simulink model "ComputedTorqueControl"  (R2020a)
settings: Solver=VariableStepAuto  StartTime=0.0  StopTime=1.5  RelTol=1e-3
values from neighbouring files (symbols this model uses):
  ADAMS_communication_interval = 0.005    [ControlsPlantTorqueControl.m]
  ADAMS_communications_per_output_step = 1    [ControlsPlantTorqueControl.m]
  ADAMS_cwd = 'C:\Users\Gowri Umesh\OneDrive\Desktop\RAJEEV_UMESH_AMORO_Report\ComputedTorqueControl'    [ControlsPlantTorqueControl.m]
  ADAMS_exec = ''    [ControlsPlantTorqueControl.m]
  ADAMS_host = 'DESKTOP-1FI5JCT'    [ControlsPlantTorqueControl.m]
  ADAMS_init = ''    [ControlsPlantTorqueControl.m]
  ADAMS_inputs = 'f1!f2'    [ControlsPlantTorqueControl.m]
  ADAMS_outputs = 'q1!q2'    [ControlsPlantTorqueControl.m]
  ADAMS_prefix = 'ControlsPlantTorqueControl'    [ControlsPlantTorqueControl.m]
  ADAMS_static = 'no'    [ControlsPlantTorqueControl.m]
  ADAMS_sysdir = 'C:\PROGRA~1\MSC~1.SOF\ADAMSS~1\2020_1\'    [ControlsPlantTorqueControl.m]
  ADAMS_time_offset = 0.0    (= 0)    [ControlsPlantTorqueControl.m]
settings Model: Creator=Gowri Umesh  LastModifiedBy=Gowri Umesh
settings DebuggingCC: AlgebraicLoopMsg=none

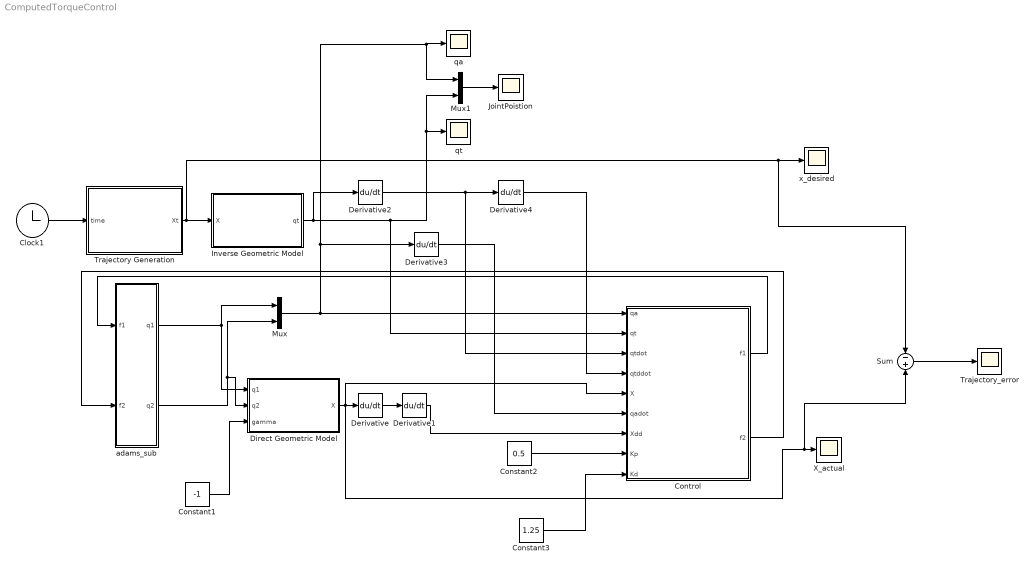
== system ComputedTorqueControl ==
  Clock1 : Clock
  Constant1 : Constant  Value=-1
  Constant2 : Constant  Value=0.5
  Constant3 : Constant  Value=1.25
  Control : MATLAB Function  TreatAsAtomicUnit=on
  Derivative{,1..4} (5 alike) : Derivative
  Direct Geometric Model : MATLAB Function  TreatAsAtomicUnit=on
  Inverse Geometric Model : MATLAB Function  TreatAsAtomicUnit=on
  JointPoistion : Scope
  Mux : Mux  Inputs=2
  Mux1 : Mux  Inputs=2
  Sum : Sum  Inputs=-+
  Trajectory Generation : MATLAB Function  TreatAsAtomicUnit=on
  Trajectory_error : Scope
  X_actual : Scope
  adams_sub : Subsystem
  qa : Scope
  qt : Scope
  x_desired : Scope
  wires:
  Sum/1 -> Trajectory_error/1
  Control/1(f1) -> adams_sub/1(f1)
  Control/2(f2) -> adams_sub/2(f2)
  Constant1/1 -> Direct Geometric Model/3(gamma)
  adams_sub/1(q1) -> Direct Geometric Model/1(q1), Mux/1
  adams_sub/2(q2) -> Mux/2, Direct Geometric Model/2(q2)
  Clock1/1 -> Trajectory Generation/1(time)
  Derivative/1 -> Derivative1/1
  Trajectory Generation/1(Xt) -> Sum/1, x_desired/1, Inverse Geometric Model/1(X)
  Mux/1 -> Mux1/1, qa/1, Derivative3/1, Control/1(qa)
  Inverse Geometric Model/1(qt) -> Derivative2/1, Mux1/2, qt/1, Control/2(qt)
  Derivative2/1 -> Control/3(qtdot), Derivative4/1
  Derivative3/1 -> Control/6(qadot)
  Direct Geometric Model/1(X) -> Control/5(X), Derivative/1, Sum/2, X_actual/1
  Derivative1/1 -> Control/7(Xdd)
  Derivative4/1 -> Control/4(qtddot)
  Constant2/1 -> Control/8(Kp)
  Constant3/1 -> Control/9(Kd)
  Mux1/1 -> JointPoistion/1

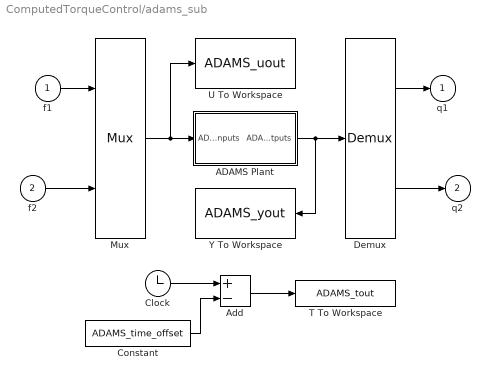
== system ComputedTorqueControl/adams_sub ==
  f1 : Inport
  f2 : Inport  Port=2
  ADAMS Plant : Subsystem  LoadFcn=|  InitFcn=clear mex  mask(Adams Plant){exevie=ADAMS_sysdir, nam_in=ADAMS_inputs, namout=ADAMS_outputs, nampre=ADAMS_prefix, outfil=ADAMS_prefix, exesol=ADAMS_exec, stat=ADAMS_static, inicmd=[ADAMS_init], exetyp=C++, comtyp=PIPE(DDE), workdir=ADAMS_cwd, ada_host=ADAMS_host, modani=batch, modsim=discrete, dft=no, simulink_lead_cosim=yes, pin_interp_order=0, pout_extrap_order=0, pin_extrap_order=0, pout_interp_order=0, dt_out=ADAMS_communication_interval, o_rate=ADAMS_communications_per_output_step, time_offset=ADAMS_time_offset, more=off}
      | %check based on dialog box setting for when setting by popup menu                                             
      | if exist('ADAMS_solver_type')                                                                                 
      |   if strcmp(ADAMS_solver_type,'C++')                                                                          
      |     set_param(gcb,'exetyp','C++');                                                                            
      |   else                                                                                                        
      |     set_param(gcb,'exetyp','Fortran');                                                                        
      |   end                                                                                                         
      | else                                                                                                          
      |   set_param(gcb,'exetyp','C++');                                                                              
      | end                                                                                                           
      | %set the mode if using acar_solver                                                                            
      | %REQUIRED HERE BECAUSE BELOW CAUSES MDLTERMINATE TO BE CALLED 2 TIMES IN MIDDLE OF SIMULATION WHEN SET IN MASK
      |                                                                                                               
      | %enable the direct feedthrough, sim mode, anim mode parameters by default                                     
      |                                                                                                               
      | if exist('set_some_params_states')                                                                            
      |                                                                                                               
      |   set_some_params_states({'dft','modsim','modani'},{'on','on','on'},'MaskEnables',gcb)                        
      |   %turn on direct feedthrough option                                                                          
      |   set_some_params_states({'dft'},{'on'},'MaskVisibilities',gcb)                                               
      |                                                                                                               
      |  end                                                                                                          
      |                                                                                                               
      |                                                                                                               
      | if exist('ADAMS_exec')                                                                                        
      |   if and(strcmp(get_param(gcb,'exesol'),'ADAMS_exec'),strcmp(ADAMS_exec,'acar_solver'))                       
      |     %set the sim mode to discrete -- only supported mode                                                      
      |     set_param(gcb,'modsim','discrete')                                                                        
      |      %turn off direct feedthrough option                                                                      
      |      set_some_params_states({'dft'},{'off'},'MaskVisibilities',gcb)                                           
      |     %set the animation mode to batch -- only supported mode                                                   
      |     set_param(gcb,'modani','batch')                                                                           
      |     %disable the direct feedthrough, sim mode, anim mode parameters                                           
      |     set_some_params_states({'modsim','modani'},{'off','off'},'MaskEnables',gcb)                               
      |   end
      |   if and(strcmp(get_param(gcb,'exesol'),'ADAMS_exec'),strcmp(ADAMS_exec,'apre_solver'))                       
      |     %set the sim mode to discrete -- only supported mode                                                      
      |     set_param(gcb,'modsim','discrete')                                                                        
      |      %turn off direct feedthrough option                                                                      
      |      set_some_params_states({'dft'},{'off'},'MaskVisibilities',gcb)                                           
      |     %set the animation mode to batch -- only supported mode                                                   
      |     set_param(gcb,'modani','batch')                                                                           
      |     %disable the direct feedthrough, sim mode, anim mode parameters                                           
      |     set_some_params_states({'modsim','modani'},{'off','off'},'MaskEnables',gcb)                               
      |   end                                                                                                  
      | end
      mask prompts: exevie "Adams install directory"; nam_in "Adams View input names"; namout "Adams View output names"; nampre "Adams model file prefix"; outfil "Output files prefix (opt.: if blank - no output)"; exesol "User executable (opt.: if blank - use standard)"; stat "Initial static simulation flag"; inicmd "Initialization commands"; exetyp "Adams Solver type"; comtyp "Interprocess option"; workdir "Adams working directory"; ada_host "Adams host"; modani "Animation mode"; modsim "Simulation mode"; dft "Direct feedthrough"; simulink_lead_cosim "Discrete Computational Order - Simulink Leads Adams"; pin_interp_order "Plant input interpolation order"; pout_extrap_order "Plant output extrapolation order"; pin_extrap_order "Plant input extrapolation order"; pout_interp_order "Plant output interpolation order"; dt_out "Communication interval"; o_rate "Number of communications per output step"; time_offset "Offset between Simulink and Adams simulation time"; more "More parameters"
      mask help: Simulate any Adams plant model either in Adams Solver form (.adm file) or in Adams View form (.cmd file)
      settings: OpenFcn=|
      | open_system(gcb,'mask')
      | if not(exist('set_some_params_states'))
      | 
      | warning('The script "set_some_params_states.m" cannot be found in the MATLAB PATH.  Cannot update the ADAMS Plant S-Function parameters.')
      | 
      | warning('Recommended action(optional):  run the Adams Controls .m file first to help choose the correct settings in the Adams S-Function block.')
      | 
      | end
      mask Help:
      | <html>
      | This S-Function represents the non-linear Adams Plant with the inputs sent to the Adams model as input #1 and Time as input #2<br>
      |  and the outputs generated by the Adams model.  See the Adams Controls documentation for more <br>
      | information.  This plant uses the following variables:<br>
      | <br>
      | <b>ADAMS_sysdir:</b> Adams installation directory<br>
      | <b>ADAMS_inputs:</b> Input variables View names vector<br>
      | <b>ADAMS_outputs :</b> Outputs variables View names vector<br>
      | <b>ADAMS_prefix:</b> ADAMS model files prefix (.adm, .cmd); also doubles as output files prefix<br>
      | <b>ADAMS_exec:</b>  Adams Solver user library or keyword (e.g., acar_solver)<br>
      | <b>ADAMS_static:</b> yes|no - initial static before Co-simulation(discrete)/Function Evaluation(continuous)<br>
      | <b>ADAMS_init:</b> Initialization commands (i.e., Adams View or Solver commands, depending on setting for Animation mode)<br>
      | <b>ADAMS_cwd:</b> Current working directory (for TCP/IP)<br>
      | <b>ADAMS_host:</b> Name of Adams server host (for TCP/IP)<br>
      | <b>ADAMS_mode:</b> Linear or non-linear (i.e., co-sim, function eval)<br>
      | <b>ADAMS_solver_type:</b> Fortran or C++ (used to set popup menu when first loaded)<br>
      | <b>ADAMS_communication_interval:</b> Time step at which Co-simulation exchange information (e.g.,0.005); also controls <br>output for continuous mode (Function Evaluation)<br>
      | <b>ADAMS_communications_per_output_step: </b>Sets Adams output rate (.res, .req, .gra) integer value (default: 1)<br>
      | <b>ADAMS_time_offset: </b>Removes this time offset from simulation time used by Adams. Adams will be sent a time value being Simulink simulation time - this value. (default: 0). Eg. if ADAMS_time_offset=2: if Simulink time=2 then Adams time = 0. Make sure that the Adams block is disabled when the Adams time is <0. If not an error will be raised. <br>
      | 
      | 
      | <br>
      | The following settings can be chosen:<br>
      | <br>
      | <b>Adams Solver type:</b>  Fortran or C++ (will also set ADAMS_solver_type)<br>
      | <b>Interprocess option:</b> Pipe(DDE), TCP/IP or DIRECT; TCP/IP can allow different machines run Adams and MATLAB<br>
      | <b>Animation mode:</b> batch (Solver, uses .adm) or interactive (View, uses .cmd)<br>
      | <b>Simulation mode:</b> discrete (Co-simulation) or continuous (Function Evaluation)<br>
      | <b>Discrete Computational Order - Simulink Lead Adams:</b> for discrete mode, chooses if Simulink leads the integration (yes) or lags (no);<br> if set to "no", can remove algebraic loop<br>
      | <b>Plant input interpolation order:</b> 0 = zero-order hold; 1 = linear (discrete mode only, where Simulink leads)<br>
      | <b>Plant output extrapolation order:</b> 0 = zero-order hold;1 = linear(discrete mode only, where Simulink leads)<br>
      | <b>Plant input extrapolation order:</b> 0 = zero-order hold; 1 = linear (discrete mode only, where Adams leads)<br>
      | <b>Plant output interpolation order:</b> 0 = zero-order hold;1 = linear(discrete mode only, where Adams leads)<br>
      | <b>Direct feedthrough:</b> yes|no - yes = Input directly effect output(continuous mode-only)<br>
      | 
      | </html>
      mask Callback exesol:
      | if exist('set_some_params_states')
      | %enable the direct feedthrough, sim mode, anim mode parameters
      | set_some_params_states({'dft','modsim','modani'},{'on','on','on'},'MaskEnables',gcb)
      | %turn on direct feedthrough option
      | set_some_params_states({'dft'},{'on'},'MaskVisibilities',gcb)
      | end
      | 
      | if exist('ADAMS_exec')
      |   if and(strcmp(get_param(gcb,'exesol'),'ADAMS_exec'),strcmp(ADAMS_exec,'acar_solver'))
      |     %set the sim mode to discrete -- only supported mode
      |     %REMOVED:  BELOW CAUSES MDLTERMINATE TO BE CALLED 2 TIMES IN MIDDLE OF SIMULATION
      |     %Now in LoadFcn callback
      |     %set_param(gcb,'modsim','discrete')
      |      %turn off direct feedthrough option
      |     set_some_params_states({'dft'},{'off'},'MaskVisibilities',gcb)
      |     %set the animation mode to batch -- only supported mode
      |     %REMOVED:  BELOW CAUSES MDLTERMINATE TO BE CALLED 2 TIMES IN MIDDLE OF SIMULATION
      |     %Now in LoadFcn callback
      |     %set_param(gcb,'modani','batch')
      |     %disable the direct feedthrough, sim mode, anim mode parameters
      |     set_some_params_states({'modsim','modani'},{'off','off'},'MaskEnables',gcb)
      |   end
      | end
      mask TypeOptions exetyp: Fortran | C++
      mask Callback exetyp:
      | if strcmp(get_param(gcb,'exetyp'),'C++')
      |     ADAMS_solver_type='C++';
      | else
      |     ADAMS_solver_type='Fortran';
      | end
      mask TypeOptions comtyp: PIPE(DDE) | TCP/IP | DIRECT
      mask Callback comtyp:
      | if exist('set_some_params_states')
      | if strcmp(get_param(gcb,'comtyp'),'PIPE(DDE)') || strcmp(get_param(gcb,'comtyp'),'DIRECT')
      |     %turn off cwd, host options
      |     set_some_params_states({'ada_host','workdir'},{'off','off'},'MaskVisibilities',gcb)
      | else%if strcmp(get_param(gcb,'modsim'),'TCP/IP')
      |     %turn on cwd, host options
      |     set_some_params_states({'ada_host','workdir'},{'on','on'},'MaskVisibilities',gcb)
      | end
      | end
      mask TypeOptions modani: batch | interactive
      mask TypeOptions modsim: discrete | continuous
      mask Callback modsim:
      | if exist('set_some_params_states')
      | if strcmp(get_param(gcb,'modsim'),'discrete')
      |      %turn off direct feedthrough option
      |     set_some_params_states({'dft'},{'off'},'MaskVisibilities',gcb)
      |     %turn on discrete co-sim type if want to see more
      |     if strcmp(get_param(gcb,'more'),'on')
      |         set_some_params_states({'simulink_lead_cosim'},{'on'},'MaskVisibilities',gcb)
      |     end
      |     if strcmp(get_param(gcb,'simulink_lead_cosim'),'yes')
      |         %turn on interpolation/extrapolation options
      |         set_some_params_states({'pin_interp_order','pout_extrap_order',},{'on','on'},'MaskVisibilities',gcb)
      |     else
      |         set_some_params_states({'pin_extrap_order','pout_interp_order'},{'on','on'},'MaskVisibilities',gcb)
      |     end
      | else%if strcmp(get_param(gcb,'modsim'),'continuous')
      |      %turn off direct feedthrough option
      |     set_some_params_states({'dft'},{'on'},'MaskVisibilities',gcb)
      |     %turn off interpolation/extrapolation options
      |     set_some_params_states({'pin_interp_order','pout_extrap_order','pin_extrap_order','pout_interp_order','simulink_lead_cosim'},{'off','off','off','off','off'},'MaskVisibilities',gcb)
      | end
      | end
      mask TypeOptions dft: no | yes
      mask TypeOptions simulink_lead_cosim: yes | no
      mask Callback simulink_lead_cosim:
      | if exist('set_some_params_states')
      | if (strcmp(get_param(gcb,'simulink_lead_cosim'),'yes') && strcmp(get_param(gcb,'modsim'),'discrete'))
      |      %turn off unused interpolate/extrapolate options
      |     set_some_params_states({'pin_extrap_order','pout_interp_order'},{'off','off'},'MaskVisibilities',gcb)
      |     %turn on used interpolate/extrapolate options
      |     set_some_params_states({'pin_interp_order','pout_extrap_order'},{'on','on'},'MaskVisibilities',gcb)
      | elseif (strcmp(get_param(gcb,'simulink_lead_cosim'),'no') && strcmp(get_param(gcb,'modsim'),'discrete'))
      |     %turn on used interpolate/extrapolate options
      |     set_some_params_states({'pin_extrap_order','pout_interp_order'},{'on','on'},'MaskVisibilities',gcb)
      |      %turn off unused interpolate/extrapolate options
      |     set_some_params_states({'pin_interp_order','pout_extrap_order'},{'off','off'},'MaskVisibilities',gcb)
      | end
      | end
      mask TypeOptions pin_interp_order: 0 | 1
      mask TypeOptions pout_extrap_order: 0 | 1
      mask TypeOptions pin_extrap_order: 0 | 1
      mask TypeOptions pout_interp_order: 0 | 1
      mask Callback more:
      | if exist('set_some_params_states')
      | if (strcmp(get_param(gcb,'more'),'on'))
      |      %turn on infrequently used options
      |     set_some_params_states({'exevie','nam_in','namout','exesol','stat','inicmd','time_offset'},{'on','on','on','on','on','on','on'},'MaskVisibilities',gcb)
      |     if strcmp(get_param(gcb,'modsim'),'discrete')
      |         set_some_params_states({'simulink_lead_cosim'},{'on'},'MaskVisibilities',gcb)
      |     end
      | elseif (strcmp(get_param(gcb,'more'),'off'))
      |     %turn off infrequently used options
      |     set_some_params_states({'exevie','nam_in','namout','exesol','stat','inicmd','time_offset'},{'off','off','off','off','off','off','off'},'MaskVisibilities',gcb)
      |     if strcmp(get_param(gcb,'modsim'),'discrete')
      |         set_some_params_states({'simulink_lead_cosim'},{'off'},'MaskVisibilities',gcb)
      |     end
      | end
      | end
      mask Display: disp( 'MSC Software' )
  Add : Sum  Inputs=+-
  Clock : Clock
  Constant : Constant  Value=ADAMS_time_offset
  Demux : Demux  Outputs=2
      settings: DisplayOption=none
  Mux : Mux  Inputs=2
  T To Workspace : ToWorkspace  VariableName=ADAMS_tout
      settings: MaxDataPoints=100000
  U To Workspace : ToWorkspace  VariableName=ADAMS_uout
      settings: MaxDataPoints=100000
  Y To Workspace : ToWorkspace  VariableName=ADAMS_yout
      settings: MaxDataPoints=100000
  q1 : Outport
  q2 : Outport  Port=2
  wires:
  Mux/1 -> ADAMS Plant/1(ADAMS inputs), U To Workspace/1
  ADAMS Plant/1(ADAMS outputs) -> Demux/1, Y To Workspace/1
  Clock/1 -> Add/1
  Constant/1 -> Add/2
  Add/1 -> T To Workspace/1
  Demux/1 -> q1/1
  Demux/2 -> q2/1
  f1/1 -> Mux/1
  f2/1 -> Mux/2

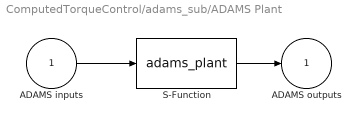
== system ComputedTorqueControl/adams_sub/ADAMS Plant ==
  ADAMS inputs : Inport
  S-Function : S-Function  StopFcn=clear mex  FunctionName=adams_plant  Parameters=exevie,exesol,stat,outfil,nampre,o_rate,nam_in,namout,dft,modsim,modani,dt_out,inicmd,exetyp,comtyp,ada_host, workdir,pin_interp_order,pout_extrap_order,pin_extrap_order,pout_interp_order,simulink_lead_cosim,time_offset  SFunctionDeploymentMode=off  EnableBusSupport=off
  ADAMS outputs : Outport  InitialOutput=0
  wires:
  ADAMS inputs/1 -> S-Function/1
  S-Function/1 -> ADAMS outputs/1

== matlab function ComputedTorqueControl/Trajectory Generation ==
  data: Xt output; time input

function Xt  = trajectory(time)

%Xa = [],Xb = [];

a1 = [-0.025;0.0125];
a2 = [0.075;-0.0375];
a4 = [0;0.3]; 
Xt = a1*time*time*time + a2*time*time + a4;
end

== matlab function ComputedTorqueControl/Direct Geometric Model ==
  data: q1 input; X output; q2 input; gamma input
function X  = DGM(q1,q2,gamma)
l = 0.3606;
d = 0.2;
E =[0 -1;1 0];

OB = [d;0];
OA = [-d;0];

AA1 = [0;q1];
BA2 = [0;q2];

A2A1 = (-BA2-OB+AA1+OA);

A2M = 0.5*(A2A1);

a = 0.5*norm(A2A1);
h =(sqrt(l^2 - a^2));
MC = gamma*(h/a)*E*A2M;

X = OB+BA2+A2M+MC;

end

== matlab function ComputedTorqueControl/Inverse Geometric Model ==
  data: X input; qt output
function qt  = IGM(X)
l = 0.3606;
d = 0.4;

x = X(1);
y = X(2);

q1 = y-(sqrt((l*l) -(x + d/2)^2));
q2 = y-(sqrt((l*l) -(x -d/2)^2));
qt = [q1;q2];
end

== matlab function ComputedTorqueControl/Control ==
  data: qa input; qt input; qtdot input; qtddot input; X input; qadot input; Xdd input; f1 output; f2 output; Kp input; Kd input

function [f1,f2] = control(qa,qt,qtdot,qtddot,X,qadot,Xdd,Kp,Kd)

d = 0.4;
m1 = 1;
m2 = 1;
mp = 3;
x = X(1);
y = X(2);

q1 = qa(1);
q2 = qa(2);

% Kp = [1.2 0;0 1.2];
% Kd = 1.2*Kp;
A = 2 *[x+d/2 y-q1;x-d/2 y-q2];
B = -2*[y-q1 0;0 y-q2];
M = [m1 0;0 m2];
c = -mp*transpose(B)*inv(transpose(A))*Xdd;


tau = M*(qtddot + Kd*(qtdot-qadot)+Kp*(qt-qa)) +c; 

f1 = tau(1);
f2 = tau(2);
end
